simulink model "Nicholos"  (R2016a)
settings: Solver=VariableStepAuto  SolverMode=SingleTasking  StartTime=0.0  StopTime=2800  RelTol=1e-3
libraries: simulink x1
settings Model: Creator=Administrator  LastModifiedBy=17513146506
settings SolverCC: ShapePreserveControl=EnableAll
settings DebuggingCC: SFUnexpectedBacktrackingDiag=error  SFNoUnconditionalDefaultTransitionDiag=error
settings SFSimCC: SimUseLocalCustomCode=on
settings RTWCC: RTWUseLocalCustomCode=on
settings GRTTargetCC: TargetLangStandard=C99 (ISO)  GeneratePreprocessorConditionals=Use local settings
settings ConfigComp: CovMetricSettings=dwe  CovHtmlReporting=off  CovSaveCumulativeToWorkspaceVar=off  CovSaveSingleToWorkspaceVar=off  CovExternalEMLEnable=on

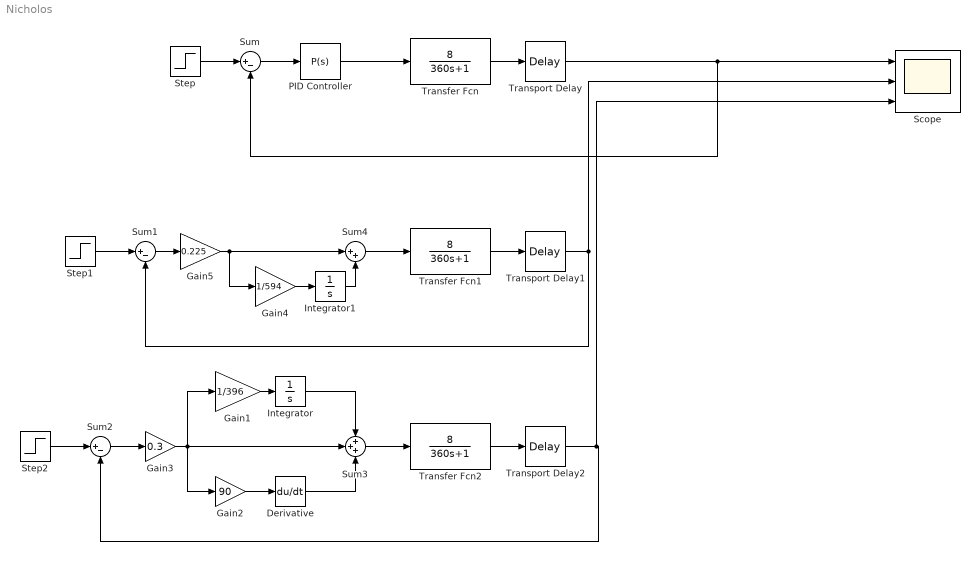
== system Nicholos ==
  Derivative : Derivative
  Gain1 : Gain  Gain=1/396
  Gain2 : Gain  Gain=90
  Gain3 : Gain  Gain=0.3
  Gain4 : Gain  Gain=1/594
  Gain5 : Gain  Gain=0.225
  Integrator : Integrator
  Integrator1 : Integrator
  PID Controller : simulink/Continuous/PID Controller  Controller=P  TimeDomain=Continuous-time  SampleTime=-1  IntegratorMethod=Forward Euler  FilterMethod=Forward Euler  Form=Parallel  UseFilter=on  ControllerParametersSource=internal  P=0.25  I=0  D=0  N=100  InitialConditionSource=internal  InitialConditionForIntegrator=0  InitialConditionForFilter=0  ExternalReset=none  LimitOutput=off  UpperSaturationLimit=inf  LowerSaturationLimit=-inf  LinearizeAsGain=on  AntiWindupMode=none  Kb=1  TrackingMode=off  Kt=1  PParamMin=[]  PParamMax=[]  IParamMin=[]  IParamMax=[]  DParamMin=[]  DParamMax=[]  NParamMin=[]  NParamMax=[]  KbParamMin=[]  KbParamMax=[]  KtParamMin=[]  KtParamMax=[]  POutMin=[]  POutMax=[]  IOutMin=[]  IOutMax=[]  DOutMin=[]  DOutMax=[]  NOutMin=[]  NOutMax=[]  KbOutMin=[]  KbOutMax=[]  KtOutMin=[]  KtOutMax=[]  IntegratorOutMin=[]  IntegratorOutMax=[]  FilterOutMin=[]  FilterOutMax=[]  SumOutMin=[]  SumOutMax=[]  SumI1OutMin=[]  SumI1OutMax=[]  SumI2OutMin=[]  SumI2OutMax=[]  SumI3OutMin=[]  SumI3OutMax=[]  SumDOutMin=[]  SumDOutMax=[]  SaturationOutMin=[]  SaturationOutMax=[]  IntegratorContinuousStateAttributes=''  IntegratorStateMustResolveToSignalObject=off  IntegratorRTWStateStorageClass=Auto  FilterContinuousStateAttributes=''  FilterStateMustResolveToSignalObject=off  FilterRTWStateStorageClass=Auto  DifferentiatorICPrevScaledInput=0  DifferentiatorOutMin=[]  DifferentiatorOutMax=[]
  Scope : Scope  NumInputPorts=3
  Step : Step  SampleTime=0
  Step1 : Step  SampleTime=0
  Step2 : Step  SampleTime=0
  Sum : Sum  Inputs=|+-
  Sum1 : Sum  Inputs=|+-
  Sum2 : Sum  Inputs=|+-
  Sum3 : Sum  Inputs=+++
  Sum4 : Sum  Inputs=|++
  Transfer Fcn : TransferFcn  Numerator=[8]  Denominator=[360 1]
  Transfer Fcn1 : TransferFcn  Numerator=[8]  Denominator=[360 1]
  Transfer Fcn2 : TransferFcn  Numerator=[8]  Denominator=[360 1]
  Transport Delay : TransportDelay  DelayTime=180
  Transport Delay1 : TransportDelay  DelayTime=180
  Transport Delay2 : TransportDelay  DelayTime=180
  wires:
  PID Controller/1 -> Transfer Fcn/1
  Transfer Fcn/1 -> Transport Delay/1
  Sum/1 -> PID Controller/1
  Step/1 -> Sum/1
  Step1/1 -> Sum1/1
  Transport Delay1/1 -> Sum1/2, Scope/2
  Transfer Fcn1/1 -> Transport Delay1/1
  Sum4/1 -> Transfer Fcn1/1
  Step2/1 -> Sum2/1
  Transport Delay2/1 -> Scope/3, Sum2/2
  Transfer Fcn2/1 -> Transport Delay2/1
  Sum2/1 -> Gain3/1
  Sum3/1 -> Transfer Fcn2/1
  Transport Delay/1 -> Scope/1, Sum/2
  Gain3/1 -> Sum3/2, Gain1/1, Gain2/1
  Integrator/1 -> Sum3/1
  Gain1/1 -> Integrator/1
  Gain2/1 -> Derivative/1
  Derivative/1 -> Sum3/3
  Gain4/1 -> Integrator1/1
  Integrator1/1 -> Sum4/2
  Sum1/1 -> Gain5/1
  Gain5/1 -> Gain4/1, Sum4/1
